simulink model "Linear_equation"  (R2023a)
settings: Solver=VariableStepAuto  StartTime=0.0  StopTime=10.0  RelTol=1e-3
undefined symbols (not defined in the file): A, B, C, D, DiscIntNeverNeededParam
libraries: simulink_extras x1, simulink x1
settings Model: Creator=tmddn  LastModifiedBy=tmddn
settings RTWCC: GPUComputeCapability=5.0

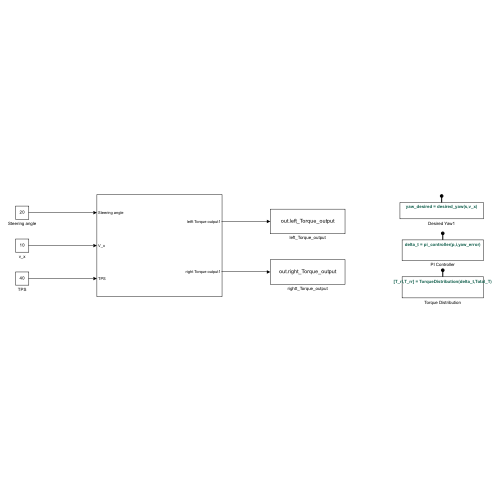
[thumbnail: Simulink's stored preview of the top-level diagram]
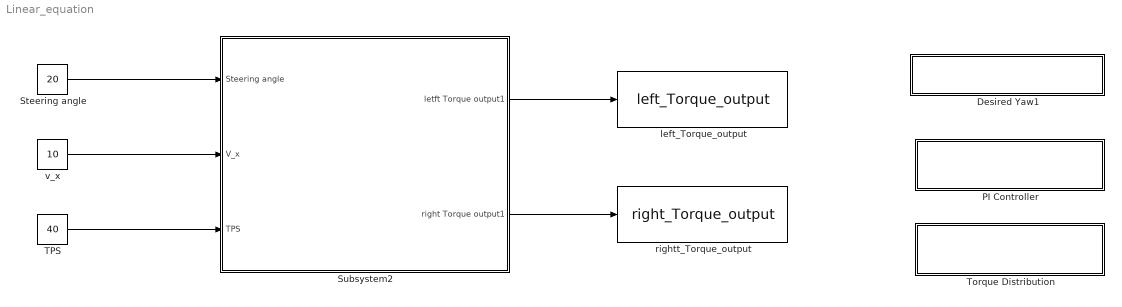
== system Linear_equation ==
  Desired Yaw1 : Subsystem  TreatAsAtomicUnit=on
  PI Controller : Subsystem  TreatAsAtomicUnit=on
  Steering angle : Constant  Value=20
  Subsystem2 : Subsystem
  TPS : Constant  Value=40
  Torque Distribution : Subsystem  TreatAsAtomicUnit=on
  left_Torque_output : ToWorkspace  VariableName=left_Torque_output  SaveFormat=Timeseries  SampleTime=-1
  rightt_Torque_output : ToWorkspace  VariableName=right_Torque_output  SaveFormat=Timeseries  SampleTime=-1
  v_x : Constant  Value=10
  wires:
  TPS/1 -> Subsystem2/3(TPS)
  Subsystem2/2(right Torque output1) -> rightt_Torque_output/1
  Steering angle/1 -> Subsystem2/1(Steering angle)
  Subsystem2/1(letft Torque output1) -> left_Torque_output/1
  v_x/1 -> Subsystem2/2(V_x)

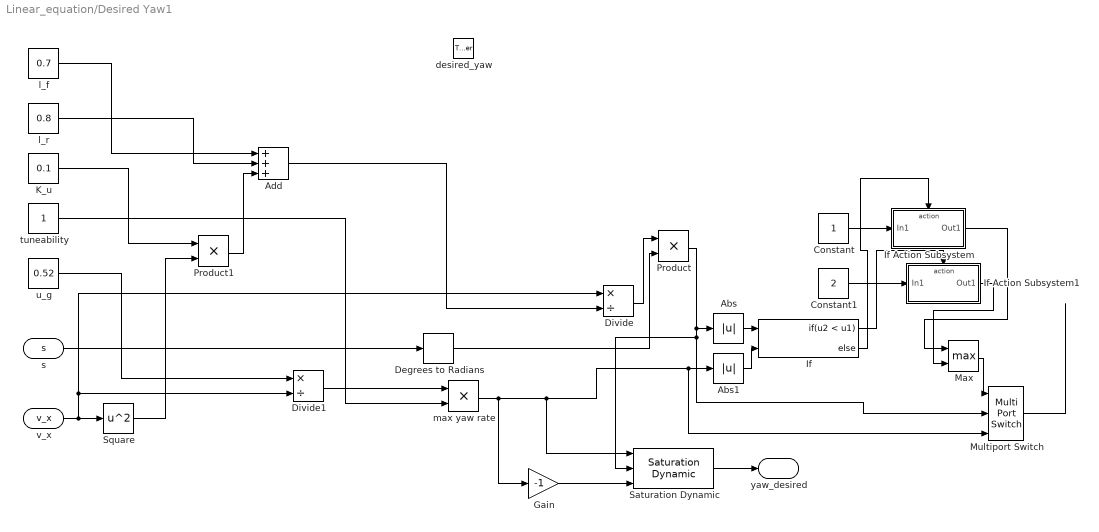
== system Linear_equation/Desired Yaw1 ==
  desired_yaw : TriggerPort  TriggerType=function-call  IsSimulinkFunction=on  FunctionName=desired_yaw  FunctionVisibility=scoped  VariantControl=(inherit)
  Abs : Abs  SaturateOnIntegerOverflow=off
  Abs1 : Abs  SaturateOnIntegerOverflow=off
  Add : Sum  Inputs=+++
  Constant : Constant
  Constant1 : Constant  Value=2
  Degrees to Radians : simulink_extras/Transformations/Degrees to Radians
  Divide : Product  Inputs=*/
  Divide1 : Product  Inputs=*/
  Gain : Gain  Gain=-1
  If : If  NumInputs=2  IfExpression=u2 < u1
  If Action Subsystem : Subsystem  TreatAsAtomicUnit=on
  If Action Subsystem1 : Subsystem  TreatAsAtomicUnit=on
  K_u : Constant  Value=0.1
  Max : MinMax  Function=max  Inputs=2
  Multiport Switch : MultiPortSwitch  Inputs=2  SaturateOnIntegerOverflow=off  InputSameDT=off
  Product : Product
  Product1 : Product
  Saturation Dynamic : simulink/Discontinuities/Saturation Dynamic  OutMin=[]  OutMax=[]  OutDataTypeStr=Inherit: Same as second input  OutDataType=fixdt(1, 16)  OutScaling=2^-10  DoSatur=off
  Square : Math  Operator=square
  l_f : Constant  Value=0.7
  l_r : Constant  Value=0.8
  max yaw rate : Product
  tuneability : Constant
  u_g : Constant  Value=0.52
  s : ArgIn  DisableCoverage=on  ArgumentName=s
  v_x : ArgIn  Port=2  ArgumentName=v_x
  yaw_desired : ArgOut  DisableCoverage=on  ArgumentName=yaw_desired
  wires:
  v_x/1 -> Divide1/2, Divide/1, Square/1
  Divide/1 -> Product/1
  s/1 -> Degrees to Radians/1
  l_f/1 -> Add/1
  l_r/1 -> Add/2
  Product1/1 -> Add/3
  K_u/1 -> Product1/1
  Square/1 -> Product1/2
  Add/1 -> Divide/2
  tuneability/1 -> max yaw rate/2
  Divide1/1 -> max yaw rate/1
  u_g/1 -> Divide1/1
  Product/1 -> Saturation Dynamic/2, Multiport Switch/2, Abs/1
  Abs/1 -> If/1
  Abs1/1 -> If/2
  max yaw rate/1 -> Gain/1, Saturation Dynamic/1, Multiport Switch/3, Abs1/1
  If Action Subsystem1/1(Out1) -> Max/2
  If/2 -> If Action Subsystem/Action
  Constant/1 -> If Action Subsystem/1(In1)
  Constant1/1 -> If Action Subsystem1/1(In1)
  If/1 -> If Action Subsystem1/Action
  If Action Subsystem/1(Out1) -> Max/1
  Max/1 -> Multiport Switch/1
  Multiport Switch/1 -> ?
  Degrees to Radians/1 -> Product/2
  Gain/1 -> Saturation Dynamic/3
  Saturation Dynamic/1 -> yaw_desired/1

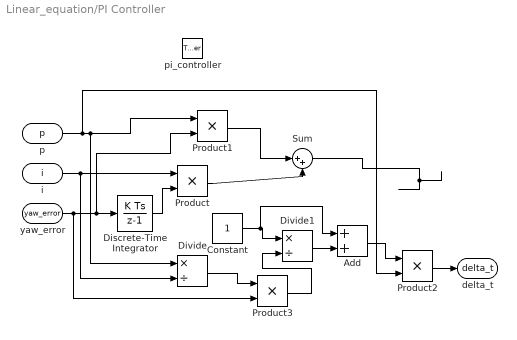
== system Linear_equation/PI Controller ==
  pi_controller : TriggerPort  TriggerType=function-call  IsSimulinkFunction=on  FunctionName=pi_controller  FunctionVisibility=scoped  VariantControl=(inherit)
  Add : Sum
  Constant : Constant
  Discrete-Time Integrator : DiscreteIntegrator  SampleTime=-1  ICPrevOutput=DiscIntNeverNeededParam  ICPrevScaledInput=DiscIntNeverNeededParam
  Divide : Product  Inputs=*/
  Divide1 : Product  Inputs=*/
  Product{,1..3} (4 alike) : Product
  Sum : Sum  Inputs=|++
  p : ArgIn  DisableCoverage=on  ArgumentName=p
  i : ArgIn  Port=2  ArgumentName=i
  yaw_error : ArgIn  Port=3  ArgumentName=yaw_error
  delta_t : ArgOut  DisableCoverage=on  ArgumentName=delta_t
  wires:
  p/1 -> Product2/2, Divide/1, Product1/1
  i/1 -> Divide/2, Product/1
  Sum/1 -> ?
  yaw_error/1 -> Product3/2, Product1/2, Discrete-Time Integrator/1
  Discrete-Time Integrator/1 -> Product/2
  Product/1 -> Sum/2
  Product1/1 -> Sum/1
  Constant/1 -> Add/1, Divide1/1
  Divide/1 -> Product3/1
  Divide1/1 -> Add/2
  Add/1 -> Product2/1
  Product2/1 -> delta_t/1
  Product3/1 -> Divide1/2

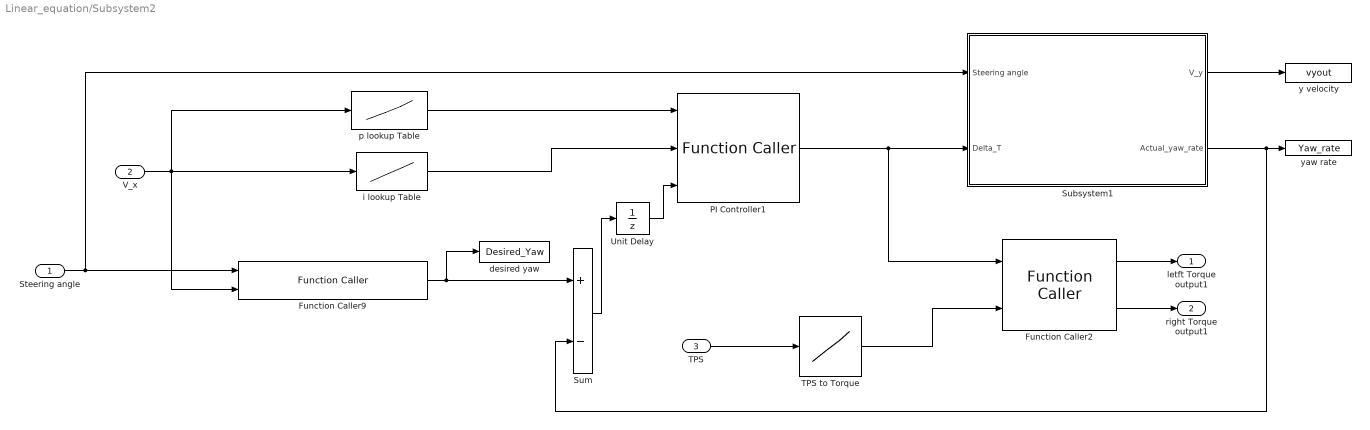
== system Linear_equation/Subsystem2 ==
  Steering angle : Inport
  V_x : Inport  Port=2
  TPS : Inport  Port=3
  Function Caller2 : FunctionCaller  FunctionPrototype=[T_rl,T_rr] = TorqueDistribution(delta_t,Total_T)  InputArgumentSpecifications=<Enter example>  OutputArgumentSpecifications=<Enter example>
  Function Caller9 : FunctionCaller  FunctionPrototype=yaw_desired = desired_yaw(s,v_x)  InputArgumentSpecifications=<Enter example>  OutputArgumentSpecifications=<Enter example>
  PI Controller1 : FunctionCaller  FunctionPrototype=delta_t = pi_controller(p,i,yaw_error)  InputArgumentSpecifications=<Enter example>  OutputArgumentSpecifications=<Enter example>
  Subsystem1 : Subsystem
  Sum : Sum  Inputs=+-
  TPS to Torque : Lookup_n-D  NumberOfTableDimensions=1  BreakpointsForDimension1=[0 10 20 30 40 50 60 70 80 90]  Table=[0 1000 3000 4000 5000 6000 7000 8000 9000 10000]  InternalRulePriority=Speed  RndMeth=Simplest
  Unit Delay : UnitDelay  SampleTime=-1  HasFrameUpgradeWarning=on
  desired yaw : ToWorkspace  VariableName=Desired_Yaw  SaveFormat=Timeseries  SampleTime=-1
  i lookup Table : Lookup_n-D  NumberOfTableDimensions=1  BreakpointsForDimension1=[7 10 13 16 19 22]  Table=[12716.7 12492.5 12040 11536.07 11058.5 13650]  InternalRulePriority=Speed  RndMeth=Simplest
  p lookup Table : Lookup_n-D  NumberOfTableDimensions=1  BreakpointsForDimension1=[7 10 13 16 19 22]  Table=[296.29 392.23 421.72 479.87 396.22 404.79]  InternalRulePriority=Speed  RndMeth=Simplest
  y velocity : ToWorkspace  VariableName=vyout  SaveFormat=Timeseries  SampleTime=-1
  yaw rate : ToWorkspace  VariableName=Yaw_rate  SaveFormat=Timeseries  SampleTime=-1
  letft Torque output1 : Outport
  right Torque output1 : Outport  Port=2
  wires:
  Function Caller9/1 -> desired yaw/1, Sum/1
  PI Controller1/1 -> Function Caller2/1, Subsystem1/2(Delta_T)
  V_x/1 -> Function Caller9/2, p lookup Table/1, i lookup Table/1
  p lookup Table/1 -> PI Controller1/1
  i lookup Table/1 -> PI Controller1/2
  Steering angle/1 -> Subsystem1/1(Steering angle), Function Caller9/1
  Sum/1 -> Unit Delay/1
  Unit Delay/1 -> PI Controller1/3
  TPS/1 -> TPS to Torque/1
  Function Caller2/1 -> letft Torque output1/1
  Function Caller2/2 -> right Torque output1/1
  TPS to Torque/1 -> Function Caller2/2
  Subsystem1/1(V_y) -> y velocity/1
  Subsystem1/2(Actual_yaw_rate) -> Sum/2, yaw rate/1

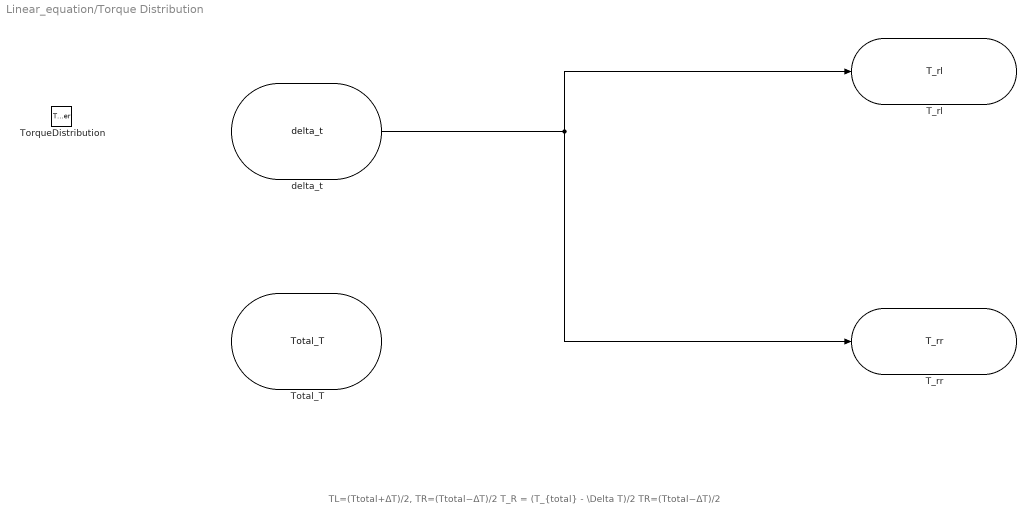
== system Linear_equation/Torque Distribution ==
  note: TL​=(Ttotal​+ΔT)/2, TR=(Ttotal−ΔT)/2 T_R = (T_{total} - \Delta T)/2 TR​=(Ttotal​−ΔT)/2
  TorqueDistribution : TriggerPort  TriggerType=function-call  IsSimulinkFunction=on  FunctionName=TorqueDistribution  FunctionVisibility=scoped  VariantControl=(inherit)
  delta_t : ArgIn  DisableCoverage=on  ArgumentName=delta_t
  Total_T : ArgIn  Port=2  ArgumentName=Total_T
  T_rl : ArgOut  DisableCoverage=on  ArgumentName=T_rl
  T_rr : ArgOut  Port=2  ArgumentName=T_rr
  wires:
  delta_t/1 -> T_rr/1, T_rl/1

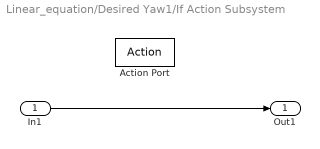
== system Linear_equation/Desired Yaw1/If Action Subsystem ==
  In1 : Inport
  Action Port : ActionPort  ActionPortLabel=else
  Out1 : Outport
  wires:
  In1/1 -> Out1/1

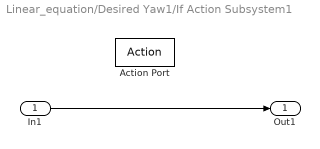
== system Linear_equation/Desired Yaw1/If Action Subsystem1 ==
  In1 : Inport
  Action Port : ActionPort  ActionPortLabel=if(u2 < u1)
  Out1 : Outport
  wires:
  In1/1 -> Out1/1

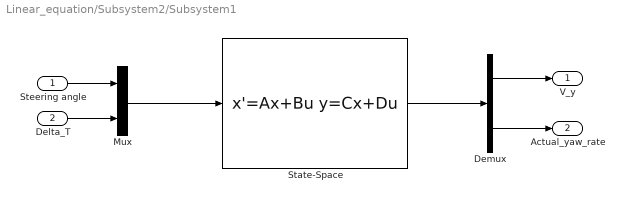
== system Linear_equation/Subsystem2/Subsystem1 ==
  Steering angle : Inport
  Delta_T : Inport  Port=2
  Demux : Demux  Outputs=2
  Mux : Mux  Inputs=2
  State-Space : StateSpace  A=A  B=B  C=C  D=D  InitialCondition=0
  V_y : Outport
  Actual_yaw_rate : Outport  Port=2
  wires:
  Mux/1 -> State-Space/1
  Delta_T/1 -> Mux/2
  State-Space/1 -> Demux/1
  Steering angle/1 -> Mux/1
  Demux/1 -> V_y/1
  Demux/2 -> Actual_yaw_rate/1
